simulink model "mobycrea_complet"  (R2019a)
settings: Solver=VariableStepAuto  StartTime=0.0  StopTime=20  RelTol=1e-3
model workspace (MAT data in the model file):
  J = 7.2e-07
  Kam = 1000
  Ke = 0.017
  Km = 0.017
  Kred = 0.0111111111111
  L = 0
  R = 11.2
settings Model: Creator=renaud  LastModifiedBy=renaud
settings ModelReferenceCC: UpdateModelReferenceTargets=Force

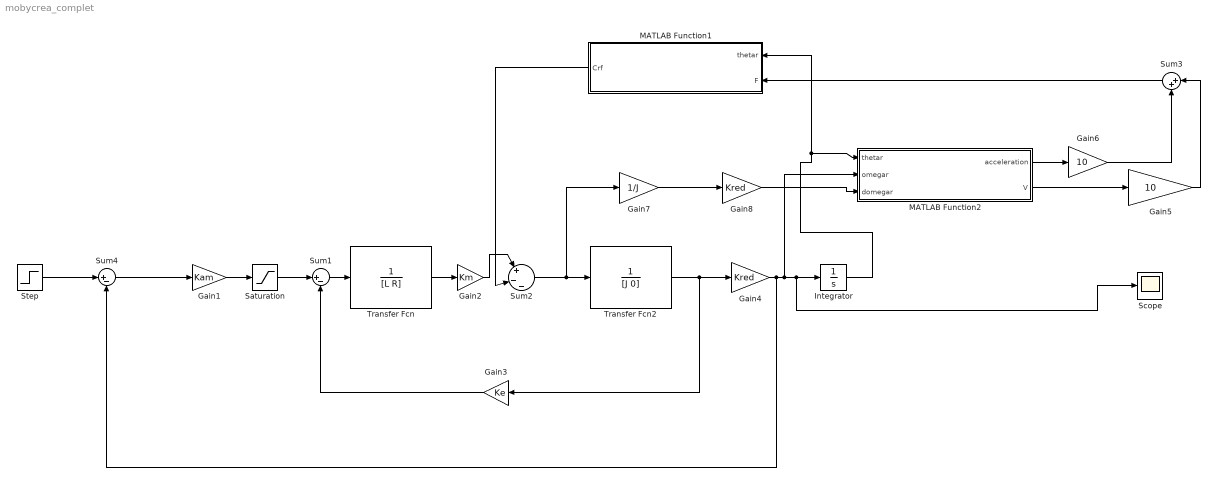
== system mobycrea_complet ==
  Gain1 : Gain  Gain=Kam
  Gain2 : Gain  Gain=Km
  Gain3 : Gain  Gain=Ke
  Gain4 : Gain  Gain=Kred
  Gain5 : Gain  Gain=10
  Gain6 : Gain  Gain=10
  Gain7 : Gain  Gain=1/J
  Gain8 : Gain  Gain=Kred
  Integrator : Integrator  InitialCondition=pi/2
  MATLAB Function1 : MATLAB Function  TreatAsAtomicUnit=on
  MATLAB Function2 : MATLAB Function  TreatAsAtomicUnit=on
  Saturation : Saturate  UpperLimit=12  LowerLimit=-12
  Scope : Scope
  Step : Step  Time=0  After=3  SampleTime=0
  Sum1 : Sum  Inputs=|+-
  Sum2 : Sum  Inputs=|+|-|-
  Sum3 : Sum  Inputs=|++
  Sum4 : Sum  Inputs=|+-
  Transfer Fcn : TransferFcn  Denominator=[L R]
  Transfer Fcn2 : TransferFcn  Denominator=[J 0]
  wires:
  Gain1/1 -> Saturation/1
  Saturation/1 -> Sum1/1
  Sum1/1 -> Transfer Fcn/1
  Gain3/1 -> Sum1/2
  Transfer Fcn/1 -> Gain2/1
  Transfer Fcn2/1 -> Gain3/1, Gain4/1
  Gain7/1 -> Gain8/1
  MATLAB Function2/1(acceleration) -> Gain6/1
  Gain4/1 -> Sum4/2, MATLAB Function2/2(omegar), Scope/1, Integrator/1
  Integrator/1 -> MATLAB Function1/1(thetar), MATLAB Function2/1(thetar)
  Gain8/1 -> MATLAB Function2/3(domegar)
  Gain2/1 -> Sum2/1
  Sum2/1 -> Gain7/1, Transfer Fcn2/1
  MATLAB Function1/1(Crf) -> Sum2/2
  MATLAB Function2/2(V) -> Gain5/1
  Gain5/1 -> Sum3/1
  Gain6/1 -> Sum3/2
  Sum3/1 -> MATLAB Function1/2(F)
  Step/1 -> Sum4/1
  Sum4/1 -> Gain1/1

== matlab function mobycrea_complet/MATLAB Function1 ==
  data: thetar input; Crf output; F input
function  Crf = calcul_couple(thetar,F)
lAB=0.036;
Crf=F*lAB*cos(thetar);

== matlab function mobycrea_complet/MATLAB Function2 ==
  data: thetar input double size=1; acceleration output double size=1; omegar input double size=1; domegar input double size=1; V output
function [acceleration,V] = calcul_acceleration(thetar,omegar,domegar)
lAB=0.036;
lBC=0.095;
theta2=pi-acos(lAB*cos(thetar)/lBC);
omega20=-lAB*sin(thetar)*omegar/(lBC*sin(theta2));
domega20=-(lAB*(cos(thetar)*omegar^2+sin(thetar)*domegar)+lBC*cos(theta2)*omega20^2)/(lBC*sin(theta2));
V=lAB*cos(thetar)*omegar+lBC*cos(theta2)*omega20;
acceleration=lAB*(cos(thetar)*domegar-sin(thetar)*omegar^2)+lBC*(cos(theta2)*domega20-sin(theta2)*omega20^2)
